simulink model "sm_ssci_hydraulic_lift_flib"  (R2024b)
settings: Solver=daessc  StartTime=0.0  StopTime=30  RelTol=1e-3  AbsTol=1e-3  EnableMultiTasking=on
PostLoadFcn:
  | warning off sm:compiler:state:UnsatisfiedDesiredTarget
  | warning off Simulink:Engine:UsingDefaultMaxStepSize
  | warning('off','sm:sli:setup:compile:SteadyStateStartNotSupported')
model workspace (MATLAB code in the model file):
  | % Units of cm
  | cyl_len = 11;
  | cyl_rOut = 1.1;
  | cyl_rInn = 1;
  | cap_len = 1;
  | 
  | pst_len = 1;
  | pst_rOut = cyl_rInn;
  | 
  | rod_len = 14;
  | rod_rOut = 0.5;
  | 
  | leg_length = 15;
  | platform_length = 25;
undefined symbols (not defined in the file or in its folder): X, Y, Z
libraries: sm_lib x21, fl_lib x14, nesl_utility x3, Multibody_Multiphysics_Lib x1, simulink x1
(part 2 of 2)

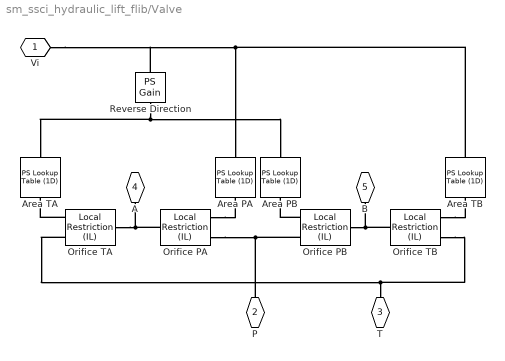
== system sm_ssci_hydraulic_lift_flib/Valve ==
  Area PA : fl_lib/Physical Signals/Lookup Tables/PS Lookup Table (1D)  x=[-x_max -x_lap 0 x_lap x_max 2*x_max]  f=[0 0 A_leak 2*A_leak A_max A_max]*1e-6  interp_method=1  extrap_method=1
  Area PB : fl_lib/Physical Signals/Lookup Tables/PS Lookup Table (1D)  x=[-x_max -x_lap 0 x_lap x_max 2*x_max]  f=[0 0 A_leak 2*A_leak A_max A_max]*1e-6  interp_method=1  extrap_method=1
  Area TA : fl_lib/Physical Signals/Lookup Tables/PS Lookup Table (1D)  x=[-x_max -x_lap 0 x_lap x_max 2*x_max]  f=[0 0 A_leak 2*A_leak A_max A_max]*1e-6  interp_method=1  extrap_method=1
  Area TB : fl_lib/Physical Signals/Lookup Tables/PS Lookup Table (1D)  x=[-x_max -x_lap 0 x_lap x_max 2*x_max]  f=[0 0 A_leak 2*A_leak A_max A_max]*1e-6  interp_method=1  extrap_method=1
  Orifice PA : fl_lib/Isothermal Liquid/Elements/Local Restriction (IL)  restriction_type=foundation.enum.restriction_type.variable  restriction_area=1e-3 m^2  min_area=1e-12 m^2  max_area=1e10 m^2  area=inf m^2  Cd=K_V  Re_c=12  pressure_recovery=simscape.enum.onoff.off
      settings: InternalSimscapePortConfiguration="{\"Bottom\":[],\"Left\":[{\"id\":\"A\",\"label\":\"A\",\"type\":\"foundation.isothermal_liquid.isothermal_liquid\"},{\"id\":\"AR\",\"label\":\"AR\",\"type\":\"input\"}],\"Right\":[{\"id\":\"B\",\"label\":\"B\",\"type\":\"foundation.isothermal_liquid.isothermal_liquid\"}],\"Top\":[]}"
      settings: LibrarySourceBlock=|
      | fl_lib/Hydraulic/Hydraulic Elements/Variable Area
      | Hydraulic Orifice
  Orifice PB : fl_lib/Isothermal Liquid/Elements/Local Restriction (IL)  restriction_type=foundation.enum.restriction_type.variable  restriction_area=1e-3 m^2  min_area=1e-12 m^2  max_area=1e10 m^2  area=inf m^2  Cd=K_V  Re_c=12  pressure_recovery=simscape.enum.onoff.off
      settings: InternalSimscapePortConfiguration="{\"Bottom\":[],\"Left\":[{\"id\":\"A\",\"label\":\"A\",\"type\":\"foundation.isothermal_liquid.isothermal_liquid\"},{\"id\":\"AR\",\"label\":\"AR\",\"type\":\"input\"}],\"Right\":[{\"id\":\"B\",\"label\":\"B\",\"type\":\"foundation.isothermal_liquid.isothermal_liquid\"}],\"Top\":[]}"
      settings: LibrarySourceBlock=|
      | fl_lib/Hydraulic/Hydraulic Elements/Variable Area
      | Hydraulic Orifice
  Orifice TA : fl_lib/Isothermal Liquid/Elements/Local Restriction (IL)  restriction_type=foundation.enum.restriction_type.variable  restriction_area=1e-3 m^2  min_area=1e-12 m^2  max_area=1e10 m^2  area=inf m^2  Cd=K_V  Re_c=12  pressure_recovery=simscape.enum.onoff.off
      settings: InternalSimscapePortConfiguration="{\"Bottom\":[],\"Left\":[{\"id\":\"A\",\"label\":\"A\",\"type\":\"foundation.isothermal_liquid.isothermal_liquid\"},{\"id\":\"AR\",\"label\":\"AR\",\"type\":\"input\"}],\"Right\":[{\"id\":\"B\",\"label\":\"B\",\"type\":\"foundation.isothermal_liquid.isothermal_liquid\"}],\"Top\":[]}"
      settings: LibrarySourceBlock=|
      | fl_lib/Hydraulic/Hydraulic Elements/Variable Area
      | Hydraulic Orifice
  Orifice TB : fl_lib/Isothermal Liquid/Elements/Local Restriction (IL)  restriction_type=foundation.enum.restriction_type.variable  restriction_area=1e-3 m^2  min_area=1e-12 m^2  max_area=1e10 m^2  area=inf m^2  Cd=K_V  Re_c=12  pressure_recovery=simscape.enum.onoff.off
      settings: InternalSimscapePortConfiguration="{\"Bottom\":[],\"Left\":[{\"id\":\"A\",\"label\":\"A\",\"type\":\"foundation.isothermal_liquid.isothermal_liquid\"},{\"id\":\"AR\",\"label\":\"AR\",\"type\":\"input\"}],\"Right\":[{\"id\":\"B\",\"label\":\"B\",\"type\":\"foundation.isothermal_liquid.isothermal_liquid\"}],\"Top\":[]}"
      settings: LibrarySourceBlock=|
      | fl_lib/Hydraulic/Hydraulic Elements/Variable Area
      | Hydraulic Orifice
  Reverse Direction : fl_lib/Physical Signals/Functions/PS Gain  gain=-1
  Vi : PMIOPort  Tag=PMCPort  Side=Left
  P : PMIOPort  Tag=PMCPort  Port=2  Side=Left
  T : PMIOPort  Tag=PMCPort  Port=3  Side=Left
  A : PMIOPort  Tag=PMCPort  Port=4  Side=Right
  B : PMIOPort  Tag=PMCPort  Port=5  Side=Right
  connections:
  Reverse Direction/RConn1 -- Area PB/LConn1 -- Area TA/LConn1
  Vi/RConn1 -- Reverse Direction/LConn1 -- Area TB/LConn1 -- Area PA/LConn1
  Orifice TA/RConn1 -- A/RConn1 -- Orifice PA/RConn1
  Orifice PA/LConn2 -- Area PA/RConn1
  P/RConn1 -- Orifice PB/LConn1 -- Orifice PA/LConn1
  Orifice PB/LConn2 -- Area PB/RConn1
  T/RConn1 -- Orifice TB/LConn1 -- Orifice TA/LConn1
  Orifice TA/LConn2 -- Area TA/RConn1
  Orifice PB/RConn1 -- B/RConn1 -- Orifice TB/RConn1
  Orifice TB/LConn2 -- Area TB/RConn1

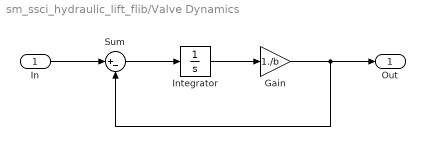
== system sm_ssci_hydraulic_lift_flib/Valve Dynamics ==
  In : Inport
  Gain : Gain  Gain=1./b
  Integrator : Integrator  InitialCondition=x_initial.*b
  Sum : Sum  Inputs=|+-  InputSameDT=on  SaturateOnIntegerOverflow=on  OutDataTypeStr=Inherit: Same as first input
  Out : Outport  VectorParamsAs1DForOutWhenUnconnected=off
  wires:
  Sum/1 -> Integrator/1
  In/1 -> Sum/1
  Integrator/1 -> Gain/1
  Gain/1 -> Sum/2, Out/1
